simulink model "Messages10"  (R2020a)
settings: Solver=VariableStepAuto  StartTime=0.0  StopTime=0.4  RelTol=1e-3
settings Model: Creator=86188  LastModifiedBy=bzhan
settings DataIOCC: ReturnWorkspaceOutputs=off
settings DebuggingCC: ArithmeticOperatorsInVariantConditions=warning
settings SFSimCC: SimUseLocalCustomCode=off  CustomCodeUndefinedFunction=UseInterfaceOnly
settings RTWCC: RTWUseLocalCustomCode=off

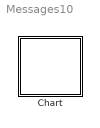
== system Messages10 ==
  Chart : Stateflow chart  TreatAsAtomicUnit=on

== stateflow chart Messages10/Chart ==
  settings: updateMethod=DISCRETE  sampleTime=0.1
  state A
    en:
    fprintf("A\n");
    M.data=3;
    send(M);
    M.data=4;
    send(M);
    M1.data=5;
    send(M1);
  state B
    en:fprintf("B\n");
    du:fprintf("B\n");
  state C
    en:fprintf("C\n");
  state D
    en:fprintf("D\n");
  (default) -> A
  A -> B : M1[M1.data==5]
  B -> C : M[M.data==4]
  C -> D : [M1.data==5]
  data: M local; M1 local
